simulink model "vrtut2"  (Simulink 7.4)
settings: Solver=ode45  StartTime=0.0  StopTime=15  RelTol=1e-3
libraries: aerospace x1, vrlib x1
Description:
  | Simulink(R) 3D Animation(TM) - Tutorial #2
  | 
  | This model represents a tutorial example, commented in the manual. See the 'Associate
  | Virtual Worlds with Simulink' chapter in the Simulink 3D Animation User's Guide.
settings Model: Creator=Straka  LastModifiedBy=Houska  CovMetricSettings=d  ExtModeTrigMode=oneshot  ExtModeArmWhenConnect=off
settings DataIOCC: SaveOutput=off  SaveTime=off  SignalLoggingName=logsOut
settings OptimizationCC: BlockReduction=off  BooleanDataType=off  InlineInvariantSignals=on  InitFltsAndDblsToZero=on
settings DebuggingCC: CheckExecutionContextPreStartOutputMsg=on  CheckExecutionContextRuntimeOutputMsg=on  SignalResolutionControl=TryResolveAllWithWarning  SolverPrmCheckMsg=none  MultiTaskDSMMsg=warning  MultiTaskCondExecSysMsg=none  StrictBusMsg=None
settings HardwareCC: TargetUnknown=on
settings ModelReferenceCC: UpdateModelReferenceTargets=IfOutOfDate
settings SFSimCC: SimGenerateEmlReport=off
settings RTWCC: IncludeERTFirstTime=on
settings GRTTargetCC: TargetFcnLib=ansi_tfl_tmw.mat

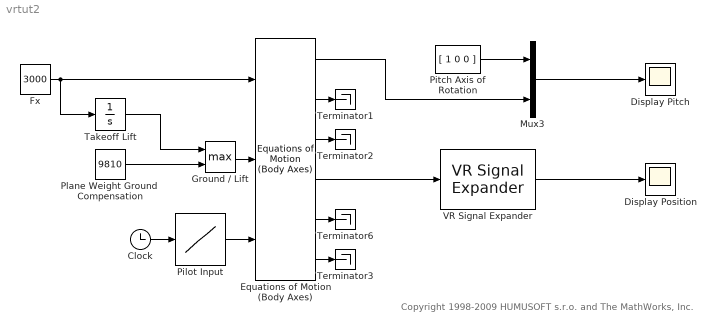
== system vrtut2 ==
  note: Copyright 1998-2009 HUMUSOFT s.r.o. and The MathWorks, Inc.
  " Equations of Motion (Body Axes)" : aerospace/3DoF Equations of Motion / Equations of Motion (Body Axes)  SystemSampleTime=-1  v_ini=0  theta_ini=0  alpha_ini=0  q_ini=0  pos_ini=[0 0]  mass=1000  Iyy=1000  g=-9.81
  Clock : Clock
      settings: Decimation=10
  Display Pitch : Scope
      settings: YMin=-2  YMax=2
  Display Position : Scope
      settings: YMax=120
  Fx : Constant  Value=3000  OutDataType=sfix(16)  OutScaling=2^0
  Ground / Lift : MinMax  Function=max  Inputs=2  OutDataType=sfix(16)  OutScaling=2^0  SaturateOnIntegerOverflow=on  InputSameDT=on
  Mux3 : Mux  Inputs=2
  Pilot Input : Lookup  InputValues=[0 1 2 8 9 15]  Table=[0 0 -20 20 0 0]  OutDataType=sfix(16)  OutScaling=2^0  SaturateOnIntegerOverflow=on
  Pitch Axis of Rotation : Constant  Value=[ 1 0 0 ]  OutDataType=sfix(16)  OutScaling=2^0
  Plane Weight Ground  Compensation : Constant  Value=9810  OutDataType=sfix(16)  OutScaling=2^0
  Takeoff Lift : Integrator  LimitOutput=on  UpperSaturationLimit=11000  LowerSaturationLimit=-Inf
  Terminator{1..3,6} (4 alike) : Terminator
  VR Signal Expander : vrlib/VR Signal Expander  SystemSampleTime=-1  outwidth=3  outidx=[3 2]
  wires:
  Pitch Axis of Rotation/1 -> Mux3/1
  " Equations of Motion (Body Axes)"/1 -> Mux3/2
  " Equations of Motion (Body Axes)"/2 -> Terminator1/1
  " Equations of Motion (Body Axes)"/3 -> Terminator2/1
  Ground / Lift/1 -> " Equations of Motion (Body Axes)"/2
  Takeoff Lift/1 -> Ground / Lift/1
  Plane Weight Ground  Compensation/1 -> Ground / Lift/2
  Clock/1 -> Pilot Input/1
  Pilot Input/1 -> " Equations of Motion (Body Axes)"/3
  Fx/1 -> " Equations of Motion (Body Axes)"/1, Takeoff Lift/1
  VR Signal Expander/1 -> Display Position/1
  Mux3/1 -> Display Pitch/1
  " Equations of Motion (Body Axes)"/6 -> Terminator3/1
  " Equations of Motion (Body Axes)"/5 -> Terminator6/1
  " Equations of Motion (Body Axes)"/4 -> VR Signal Expander/1
